simulink model "wk2_twotank_model"  (R2020a)
settings: Solver=VariableStepAuto  StartTime=0.0  StopTime=tsim  RelTol=1e-3
values from neighbouring files (symbols this model uses):
  flowgain = 0.0676    [wk2_twotank.m]
  flowgain2 = 0.057    [wk2_twotank.m]
  Kbot = 14.844    [twotank_RL.m]    (also in wk2_twotank.m)
  Ki = 0.001253    [twotank_RL.m]    (also in wk2_twotank.m = 0.004)
  Kp = 0.18164    [twotank_RL.m]    (also in wk2_twotank.m = 0.6)
  Ktop = 17.533    [twotank_RL.m]    (also in wk2_twotank.m)
  T = 100    [twotank_RL.m]    (also in wk2_twotank.m)
  valvegain = 8.9172    [wk2_twotank.m]
libraries: simulink x1
settings Model: Creator=nash  LastModifiedBy=nash
settings DataIOCC: ReturnWorkspaceOutputs=off

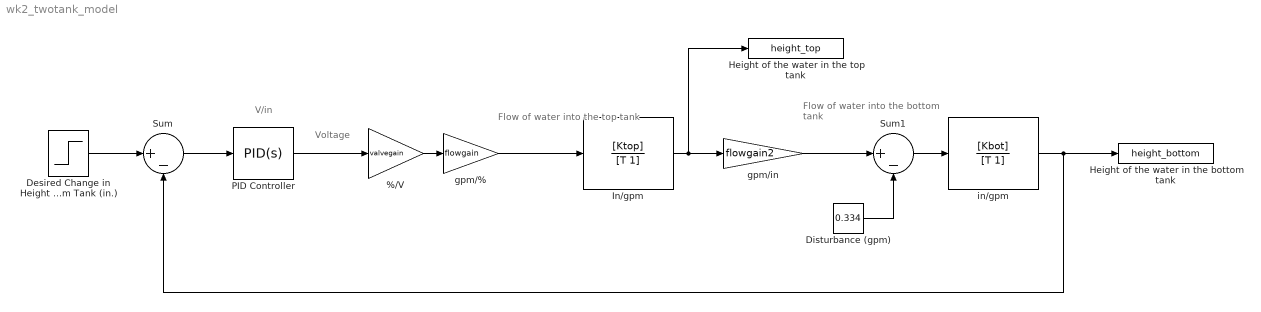
== system wk2_twotank_model ==
  note: V/in
  note: Voltage
  note: Flow of water into the top tank
  note: Flow of water into the bottom tank
  %/V : Gain  Gain=valvegain
  Desired Change in Height of Bottom Tank (in.) : Step  Time=10  After=0  SampleTime=0
  Disturbance (gpm) : Constant  Value=0.334
  Height of the water in the bottom tank : ToWorkspace  VariableName=height_bottom  SampleTime=-1
  Height of the water in the top tank : ToWorkspace  VariableName=height_top  SampleTime=-1
  In/gpm : TransferFcn  Numerator=[Ktop]  Denominator=[T 1]
  PID Controller : simulink/Continuous/PID Controller  Controller=PID  Form=Parallel  TimeDomain=Continuous-time  UseExternalTs=off  SampleTime=-1  IntegratorMethod=Forward Euler  FilterMethod=Forward Euler  ControllerParametersSource=internal  P=Kp  I=Ki  D=0  UseFilter=on  N=100  TunerSelectOption=Transfer Function Based (PID Tuner App)  InitialConditionSource=internal  InitialConditionForIntegrator=0  InitialConditionForFilter=0  DifferentiatorICPrevScaledInput=0  ExternalReset=none  TrackingMode=off  Kt=1  LimitOutput=off  UpperSaturationLimit=inf  LowerSaturationLimit=-inf  LinearizeAsGain=on  AntiWindupMode=none  Kb=1  POutMin=[]  POutMax=[]  IOutMin=[]  IOutMax=[]  DOutMin=[]  DOutMax=[]  NOutMin=[]  NOutMax=[]  SumOutMin=[]  SumOutMax=[]  SaturationOutMin=[]  SaturationOutMax=[]  PParamMin=[]  PParamMax=[]  IParamMin=[]  IParamMax=[]  DParamMin=[]  DParamMax=[]  NParamMin=[]  NParamMax=[]  KbParamMin=[]  KbParamMax=[]  KtParamMin=[]  KtParamMax=[]  KbOutMin=[]  KbOutMax=[]  KtOutMin=[]  KtOutMax=[]  IntegratorOutMin=[]  IntegratorOutMax=[]  FilterOutMin=[]  FilterOutMax=[]  SumI1OutMin=[]  SumI1OutMax=[]  SumI2OutMin=[]  SumI2OutMax=[]  SumI3OutMin=[]  SumI3OutMax=[]  SumI4OutMin=[]  SumI4OutMax=[]  SumDOutMin=[]  SumDOutMax=[]  DifferentiatorOutMin=[]  DifferentiatorOutMax=[]  FilterDiffOutCoefMin=[]  FilterDiffOutCoefMax=[]  ReciprocalOutMin=[]  ReciprocalOutMax=[]  SumDenOutMin=[]  SumDenOutMax=[]  SumNumOutMin=[]  SumNumOutMax=[]  DivideOutMin=[]  DivideOutMax=[]  UdiffTsProdOutMin=[]  UdiffTsProdOutMax=[]  NTsProdOutMin=[]  NTsProdOutMax=[]  UintegralTsProdOutMin=[]  UintegralTsProdOutMax=[]  UngainTsProdOutMin=[]  UngainTsProdOutMax=[]  IntegratorContinuousStateAttributes=''  IntegratorStateMustResolveToSignalObject=off  IntegratorRTWStateStorageClass=Auto  FilterContinuousStateAttributes=''  FilterStateMustResolveToSignalObject=off  FilterRTWStateStorageClass=Auto  ParallelPVariant=InternalParameters  IdealPVariant=Disabled  IVariant=InternalParameters  DVariant=InternalParameters  IntegratorVariant=Continuous  SatVariant=Disabled  AWVariant=Passthrough  PCopyVariant=Disabled  TRVariant=Disabled  FdbkBlocksVariant=Forward  IdealPFdbkVariant=Disabled  SatFdbkVariant=Disabled  DerivativeFilterVariant=ContFilter  NVariant=InternalParameters  NCopyVariant=Disabled  FilterICVariant=InternalICsFilter  IntegratorICVariant=InternalICs  ExternalResetVariant=Disabled  TRSumVariant=Passthrough  SumFdbkVariant=Disabled  SumVariant=Sum_PID  TsampFilterVariant=InternalTs  TsampNgainVariant=Passthrough  TsampIntegralVariant=Passthrough
  Sum : Sum  Inputs=|+-
  Sum1 : Sum  Inputs=|+-
  gpm/% : Gain  Gain=flowgain
  gpm/in : Gain  Gain=flowgain2
  in/gpm : TransferFcn  Numerator=[Kbot]  Denominator=[T 1]
  wires:
  %/V/1 -> gpm/%/1
  gpm/%/1 -> In/gpm/1
  In/gpm/1 -> Height of the water in the top tank/1, gpm/in/1
  in/gpm/1 -> Sum/2, Height of the water in the bottom tank/1
  Sum/1 -> PID Controller/1
  PID Controller/1 -> %/V/1
  Sum1/1 -> in/gpm/1
  gpm/in/1 -> Sum1/1
  Disturbance (gpm)/1 -> Sum1/2
  Desired Change in Height of Bottom Tank (in.)/1 -> Sum/1
